simulink model "Q2_simulation"  (R2021a)
settings: Solver=VariableStepAuto  StartTime=0.0  StopTime=10.0  RelTol=1e-3
values from neighbouring files (symbols this model uses):
  A = [0           0               1                 0 ... (first row only)    [Q1_1.m]    (also in Q1_2.m; Q1_3.m)
  B = [0 0 1/mc 1/(L*mc)]'    [Q1_1.m]    (also in Q1_2.m; Q1_3.m)
undefined symbols (not defined in the file or in its folder): C
settings Model: Creator=Tushar  LastModifiedBy=Tushar

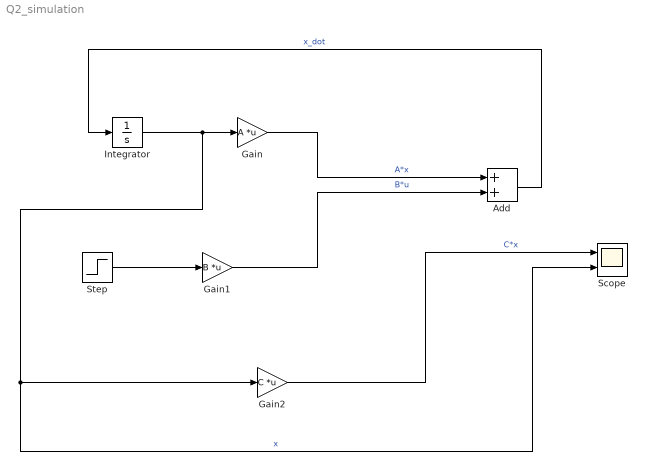
== system Q2_simulation ==
  Add : Sum
  Gain : Gain  Gain=A  Multiplication=Matrix(K*u)
  Gain1 : Gain  Gain=B  Multiplication=Matrix(K*u)
  Gain2 : Gain  Gain=C  Multiplication=Matrix(K*u)
  Integrator : Integrator  InitialCondition=[0 0 (10*pi)/180 0]
  Scope : Scope  NumInputPorts=2
  Step : Step  Time=0  SampleTime=0
  wires:
  Integrator/1 -> Scope/2, Gain2/1, Gain/1  "x"
  Add/1 -> Integrator/1  "x_dot"
  Gain/1 -> Add/1  "A*x"
  Gain1/1 -> Add/2  "B*u"
  Gain2/1 -> Scope/1  "C*x"
  Step/1 -> Gain1/1
